simulink model "wheelControl"  (R2014a)
settings: Solver=ode45  StartTime=0.0  StopTime=10.0  RelTol=1e-3
values from neighbouring files (symbols this model uses):
  B1 = 1    [FinalProject.m]
  Bm = 1    [FinalProject.m]
  coeffs = flip(tMat \ varMat)    [CalcSpline.m]    (also in CalcTrajectory.m = [ax, ay]; FinalProject.m = rightCoeffs(1,:))
  g1 = 1    [FinalProject.m]
  J1 = 1    [FinalProject.m]
  Jm = 1    [FinalProject.m]
  L1 = 1    [FinalProject.m]
  m1 = 1    [FinalProject.m]
  N = 1    [FinalProject.m]
libraries: simulink x2
settings Model: Creator=collinsjm  LastModifiedBy=beaverl

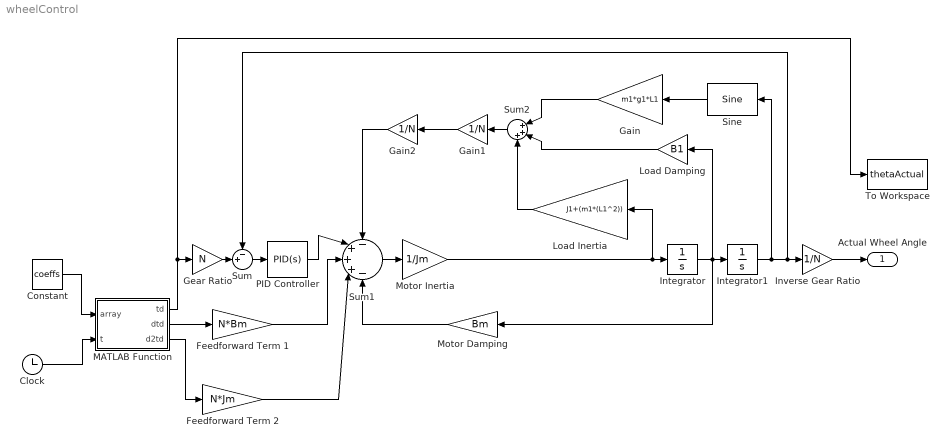
== system wheelControl ==
  Clock : Clock
  Constant : Constant  Value=coeffs
  Feedforward Term 1 : Gain  Gain=N*Bm
  Feedforward Term 2 : Gain  Gain=N*Jm
  Gain : Gain  Gain=m1*g1*L1
  Gain1 : Gain  Gain=1/N
  Gain2 : Gain  Gain=1/N
  Gear Ratio : Gain  Gain=N
  Integrator : Integrator
  Integrator1 : Integrator
  Inverse Gear Ratio : Gain  Gain=1/N
  Load Damping : Gain  Gain=B1
  Load Inertia : Gain  Gain=J1+(m1*(L1^2))
  MATLAB Function : MATLAB Function  TreatAsAtomicUnit=on
  Motor Damping : Gain  Gain=Bm
  Motor Inertia : Gain  Gain=1/Jm
  PID Controller : simulink/Continuous/PID Controller  Controller=PID  TimeDomain=Continuous-time  SampleTime=1  IntegratorMethod=Forward Euler  FilterMethod=Forward Euler  Form=Parallel  P=1  I=1  D=0  N=100  InitialConditionSource=internal  InitialConditionForIntegrator=0  InitialConditionForFilter=0  ExternalReset=none  LimitOutput=off  UpperSaturationLimit=inf  LowerSaturationLimit=-inf  LinearizeAsGain=on  AntiWindupMode=none  Kb=1  TrackingMode=off  Kt=1  PParamMin=[]  PParamMax=[]  IParamMin=[]  IParamMax=[]  DParamMin=[]  DParamMax=[]  NParamMin=[]  NParamMax=[]  KbParamMin=[]  KbParamMax=[]  KtParamMin=[]  KtParamMax=[]  POutMin=[]  POutMax=[]  IOutMin=[]  IOutMax=[]  DOutMin=[]  DOutMax=[]  NOutMin=[]  NOutMax=[]  KbOutMin=[]  KbOutMax=[]  KtOutMin=[]  KtOutMax=[]  IntegratorOutMin=[]  IntegratorOutMax=[]  FilterOutMin=[]  FilterOutMax=[]  SumOutMin=[]  SumOutMax=[]  SumI1OutMin=[]  SumI1OutMax=[]  SumI2OutMin=[]  SumI2OutMax=[]  SumI3OutMin=[]  SumI3OutMax=[]  SumDOutMin=[]  SumDOutMax=[]  SaturationOutMin=[]  SaturationOutMax=[]  IntegratorContinuousStateAttributes=''  IntegratorStateMustResolveToSignalObject=off  IntegratorRTWStateStorageClass=Auto  FilterContinuousStateAttributes=''  FilterStateMustResolveToSignalObject=off  FilterRTWStateStorageClass=Auto
  Sine : simulink/Lookup Tables/Sine  Formula=sin(2*pi*u)  NumDataPoints=(2^5)+1  OutputWordLength=16  InternalRulePriority=Speed
  Sum : Sum  Inputs=-+|
  Sum1 : Sum  Inputs=-+++-
  Sum2 : Sum  Inputs=|+++
  To Workspace : ToWorkspace  VariableName=thetaActual  SaveFormat=Timeseries  SampleTime=-1
  Actual Wheel Angle : Outport
  wires:
  Constant/1 -> MATLAB Function/1(array)
  Clock/1 -> MATLAB Function/2(t)
  MATLAB Function/1(td) -> To Workspace/1, Gear Ratio/1
  Gear Ratio/1 -> Sum/2
  Sum/1 -> PID Controller/1
  Sum1/1 -> Motor Inertia/1
  Motor Inertia/1 -> Load Inertia/1, Integrator/1
  Integrator/1 -> Load Damping/1, Integrator1/1, Motor Damping/1
  PID Controller/1 -> Sum1/2
  Motor Damping/1 -> Sum1/5
  Integrator1/1 -> Sine/1, Inverse Gear Ratio/1, Sum/1
  Sine/1 -> Gain/1
  Gain/1 -> Sum2/1
  Load Damping/1 -> Sum2/2
  Load Inertia/1 -> Sum2/3
  Sum2/1 -> Gain1/1
  Gain1/1 -> Gain2/1
  Gain2/1 -> Sum1/1
  MATLAB Function/2(dtd) -> Feedforward Term 1/1
  Feedforward Term 1/1 -> Sum1/3
  MATLAB Function/3(d2td) -> Feedforward Term 2/1
  Feedforward Term 2/1 -> Sum1/4
  Inverse Gear Ratio/1 -> Actual Wheel Angle/1

== matlab function wheelControl/MATLAB Function ==
  data: array input; td output; t input; dtd output; d2td output
function [td,dtd,d2td] = thetaD(array,t)
%#codegen

dtd=0;
d2td=0;
td=polyval(array,t);
for i=1:length(array)-1
    dtd=dtd+(i*array(i+1)*(t^(i-1)));
    if not(i==1)
        d2td=d2td+((i-1)*i*array(i+1)*(t^(i-2)));
    end
end
